simulink model "robot_simulation"  (R2025a)
settings: Solver=VariableStepAuto  StartTime=0.0  StopTime=50  FixedStep=0.01  MaxStep=0.1  RelTol=1e-3
settings Model: Creator=davrahnpaur  LastModifiedBy=davrahnpaur

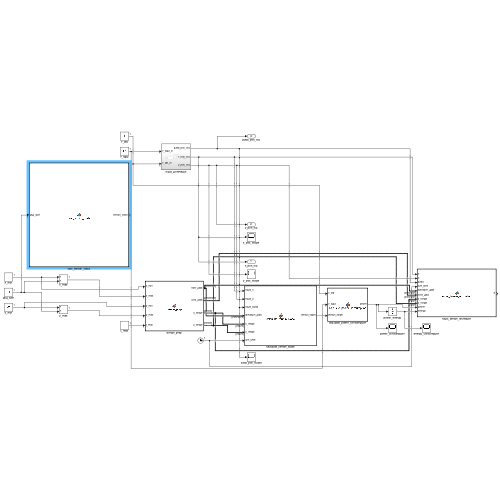
[thumbnail: Simulink's stored preview of the top-level diagram]
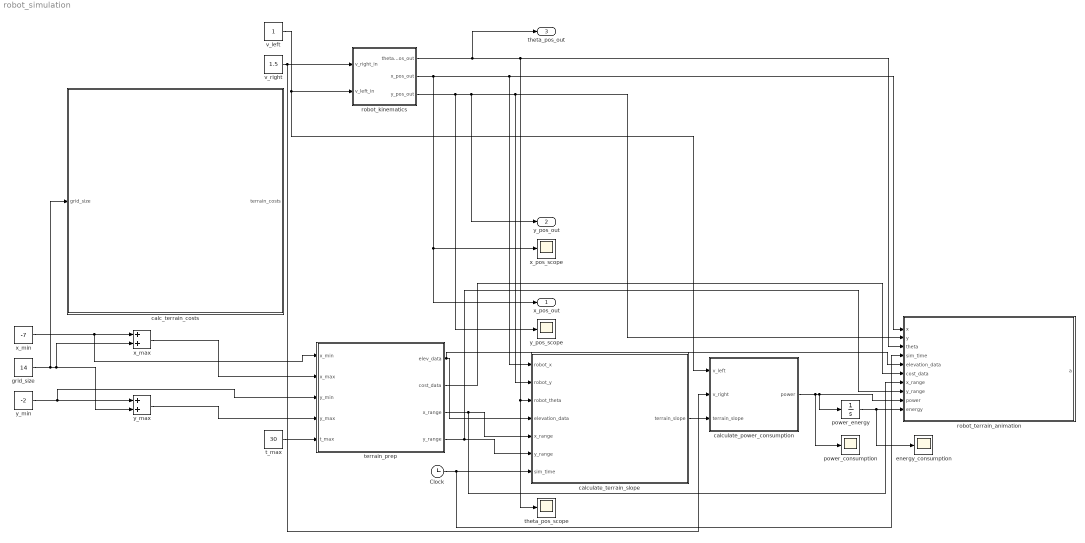
== system robot_simulation ==
  Clock : Clock
  calc_terrain_costs : MATLAB Function  TreatAsAtomicUnit=on
  calculate_power_consumption : MATLAB Function  TreatAsAtomicUnit=on
  calculate_terrain_slope : MATLAB Function  TreatAsAtomicUnit=on  SystemSampleTime=0.01
  energy_consumption : Scope
      settings: ActiveDisplayYMinimum=-15.735326881390064  ActiveDisplayYMaximum=141.6179419325106  DataLoggingVariableName=ScopeData4
  grid_size : Constant  Value=14
  power_consumption : Scope
      settings: ActiveDisplayYMinimum=1.5743115904386631  ActiveDisplayYMaximum=3.4296984826344525  DataLoggingVariableName=ScopeData3
  power_energy : Integrator
  robot_kinematics : Subsystem
  robot_terrain_animation : MATLAB Function  TreatAsAtomicUnit=on  SystemSampleTime=0.5
  t_max : Constant  Value=30
  terrain_prep : MATLAB Function  TreatAsAtomicUnit=on
  theta_pos_scope : Scope
      settings: ActiveDisplayYMinimum=-1  ActiveDisplayYMaximum=1
  v_left : Constant
  v_right : Constant  Value=1.5
  x_max : Sum
  x_min : Constant  Value=-7
  x_pos_scope : Scope
      settings: ActiveDisplayYMinimum=-1  ActiveDisplayYMaximum=1
  y_max : Sum
  y_min : Constant  Value=-2
  y_pos_scope : Scope
      settings: ActiveDisplayYMinimum=-1  ActiveDisplayYMaximum=1  DataLoggingVariableName=ScopeData2
  x_pos_out : Outport
  y_pos_out : Outport  Port=2
  theta_pos_out : Outport  Port=3
  wires:
  power_energy/1 -> robot_terrain_animation/10(energy), energy_consumption/1
  calculate_terrain_slope/1(terrain_slope) -> calculate_power_consumption/3(terrain_slope)
  calculate_power_consumption/1(power) -> power_energy/1, robot_terrain_animation/9(power), power_consumption/1
  Clock/1 -> calculate_terrain_slope/7(sim_time), robot_terrain_animation/4(sim_time)
  terrain_prep/4(y_range) -> calculate_terrain_slope/6(y_range), robot_terrain_animation/8(y_range)
  terrain_prep/3(x_range) -> calculate_terrain_slope/5(x_range), robot_terrain_animation/7(x_range)
  terrain_prep/2(cost_data) -> robot_terrain_animation/6(cost_data)
  terrain_prep/1(elev_data) -> calculate_terrain_slope/4(elevation_data), robot_terrain_animation/5(elevation_data)
  t_max/1 -> terrain_prep/5(t_max)
  robot_kinematics/3(y_pos_out) -> calculate_terrain_slope/2(robot_y), robot_terrain_animation/2(y), y_pos_out/1, y_pos_scope/1
  x_min/1 -> x_max/1, terrain_prep/1(x_min)
  robot_kinematics/1(theta_pos_out) -> calculate_terrain_slope/3(robot_theta), theta_pos_scope/1, robot_terrain_animation/3(theta), theta_pos_out/1
  x_max/1 -> terrain_prep/2(x_max)
  grid_size/1 -> y_max/2, x_max/2, calc_terrain_costs/1(grid_size)
  y_max/1 -> terrain_prep/4(y_max)
  v_right/1 -> robot_kinematics/1(v_right_in), calculate_power_consumption/2(v_right)
  robot_kinematics/2(x_pos_out) -> x_pos_out/1, x_pos_scope/1, calculate_terrain_slope/1(robot_x), robot_terrain_animation/1(x)
  y_min/1 -> y_max/1, terrain_prep/3(y_min)
  v_left/1 -> robot_kinematics/2(v_left_in), calculate_power_consumption/1(v_left)

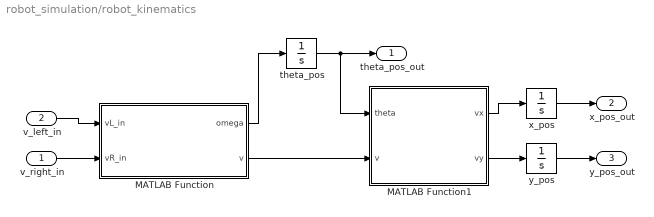
== system robot_simulation/robot_kinematics ==
  v_right_in : Inport
  v_left_in : Inport  Port=2
  MATLAB Function : MATLAB Function  TreatAsAtomicUnit=on
  MATLAB Function1 : MATLAB Function  TreatAsAtomicUnit=on
  theta_pos : Integrator
  x_pos : Integrator  ContinuousStateAttributes='x_position'
  y_pos : Integrator  ContinuousStateAttributes='y_position'
  theta_pos_out : Outport
  x_pos_out : Outport  Port=2
  y_pos_out : Outport  Port=3
  wires:
  x_pos/1 -> x_pos_out/1
  MATLAB Function1/2(vy) -> y_pos/1
  MATLAB Function1/1(vx) -> x_pos/1
  v_left_in/1 -> MATLAB Function/1(vL_in)
  v_right_in/1 -> MATLAB Function/2(vR_in)
  theta_pos/1 -> MATLAB Function1/1(theta), theta_pos_out/1
  y_pos/1 -> y_pos_out/1
  MATLAB Function/2(v) -> MATLAB Function1/2(v)
  MATLAB Function/1(omega) -> theta_pos/1

== matlab function robot_simulation/robot_kinematics/MATLAB Function ==
  data: vL_in input; omega output; vR_in input; v output
function [omega,v] = velocity_transform(vL_in,vR_in)

    omega = (vR_in-vL_in)/2;
    v = (vR_in+vL_in)/2;
end

== matlab function robot_simulation/robot_terrain_animation ==
  data: x input; y input; theta input; a output; sim_time input; elevation_data input; cost_data input; x_range input; y_range input; power input; energy input
function a = robot_terrain_animation(x, y, theta, sim_time, elevation_data, cost_data, x_range, y_range, power, energy)
%#codegen
    persistent trail_x trail_y X_grid Y_grid
    
    % Initialize grid (do once)
    if isempty(X_grid)
        [X_grid, Y_grid] = meshgrid(x_range, y_range);
        trail_x = [];
        trail_y = [];
    end
    
    % Calculate current terrain time slice
    time_index = max(1, min(sim_time+1, size(elevation_data,3)));
    current_elevation = elevation_data(:,:,time_index);
    current_cost = cost_data(:,:,time_index);
    
    % Clear and redraw
    cla;
    
    % Draw terrain background
    % Cost as heatmap background
    imagesc(x_range, y_range, current_cost);
    hold on;
    
    % Elevation as contour lines
    contour(x_range, y_range, current_elevation, 'k-', 'LineWidth', 0.5);
    
    % Your existing robot visualization
    plot(x, y, 'ro', 'MarkerSize', 10, 'MarkerFaceColor', 'red');
    
    % Robot heading arrow
    arrow_length = 0.5;
    arrow_x = [x, x + arrow_length*cos(theta)];
    arrow_y = [y, y + arrow_length*sin(theta)];
    plot(arrow_x, arrow_y, 'b-', 'LineWidth', 3);
    
    % Trail
    trail_x = [trail_x, x];
    trail_y = [trail_y, y];
    plot(trail_x, trail_y, 'g--', 'LineWidth', 2);
    
    % Formatting
    axis equal;
    xlim([x_range(1), x_range(end)]);
    ylim([y_range(1), y_range(end)]);
    colorbar;  % Show cost scale
    title(sprintf('Time: %.1f s | Power: %.1f W | Energy: %.1f J', sim_time, power, energy));
    
    drawnow;
    a = 0;
end

== matlab function robot_simulation/robot_kinematics/MATLAB Function1 ==
  data: theta input; vx output; v input; vy output
function [vx,vy] = velocity_transform2(theta,v)
   vx = v*cos(theta);
   vy = v*sin(theta);
end

== matlab function robot_simulation/terrain_prep ==
  data: elev_data output; cost_data output; x_range output; y_range output; x_min input; x_max input; y_min input; y_max input; t_max input
function [elev_data, cost_data, x_range, y_range] = terrain_prep(x_min,x_max,y_min,y_max,t_max)
    % Define spatial grid - these should match your animation axis limits
    num_x = (x_max - x_min) + 1;
    num_y = (y_max - y_min) + 1;
    x_range = linspace(x_min, x_max, num_x);
    y_range = linspace(y_min, y_max, num_y);
    
    % Time parameters
    time_steps = t_max + 1;  % Number of terrain snapshots
    
    % Initialize terrain arrays
    elev_data = zeros(length(y_range), length(x_range), time_steps);
    cost_data = zeros(length(y_range), length(x_range), time_steps);
    
    % Create example terrain that changes over time
    [x_grid, y_grid] = meshgrid(x_range, y_range);
    
    for t = 1:time_steps
        time_factor = t-1;
        
        % Example elevation: moving sine wave
        elev_data(:,:,t) = 2 * sin(0.3 * x_grid + 0.1 * time_factor) .* cos(0.2 * y_grid);
        
        % Example cost: moving high-cost regions
        cost_data(:,:,t) = 1 + 2 * exp(-((x_grid - 5 - time_factor/3).^2 + (y_grid - 2).^2) / 4);
    end
end

== matlab function robot_simulation/calculate_power_consumption ==
  data: v_left input; power output; v_right input; terrain_slope input
function power = calculate_power_consumption(v_left, v_right, terrain_slope)

    % Base power consumption (flat terrain)
    base_power_left = abs(v_left);% * 10;   % 10 watts per m/s
    base_power_right = abs(v_right);% * 10; % 10 watts per m/s
    
    % Slope effect multiplier
    % Positive slope (uphill) increases power, negative (downhill) decreases it
    slope_multiplier = 1 + terrain_slope * 0.5;  % 50% more power per unit slope
    slope_multiplier = max(0.1, slope_multiplier); % Minimum 10% power (even downhill)
    
    % Total power consumption
    power = (base_power_left + base_power_right) * slope_multiplier;

end

== matlab function robot_simulation/calc_terrain_costs ==
  data: grid_size input; terrain_costs output
function terrain_costs = calc_terrain_costs(grid_size)
    % Define grid dimensions
    
    % Define terrain types and their properties, INCLUDING COSTS
    terrain_types = {
        struct('name', 'Grass', 'color', [0.3 0.6 0.2], 'cost', 1.0);     % Green, low cost
        struct('name', 'Sand', 'color', [0.9 0.8 0.5], 'cost', 2.0);      % Light Brown/Yellow, moderate cost
        struct('name', 'Mud', 'color', [0.5 0.3 0.1], 'cost', 3.0);       % Dark Brown, higher cost
        struct('name', 'Road', 'color', [0.6 0.6 0.6], 'cost', 0.5);      % Grey, very low cost (fast)
        struct('name', 'Water', 'color', [0.2 0.4 0.8], 'cost', inf);     % Blue, impassable
        struct('name', 'Forest', 'color', [0.1 0.4 0.1], 'cost', 2.5);    % Darker Green, moderate-high cost
    };
    num_terrain_types = length(terrain_types);
    
    terrain_grid = zeros(grid_size, grid_size);
    
    % --- Initial Random Terrain Generation ---
    % Assign a random terrain type to each cell in the grid
    for i = 1:grid_size
        for j = 1:grid_size
            terrain_grid(i, j) = randi(num_terrain_types);
        end
    end
    
    % --- Terrain Smoothing (to create grouped regions) ---
    num_smoothing_iterations = 5;
    for iter = 1:num_smoothing_iterations
        new_terrain_grid = terrain_grid; % Create a copy to store updates for this iteration
        for i = 1:grid_size
            for j = 1:grid_size
                neighbors = [];
                % Check 8-directional neighbors
                for dx = -1:1
                    for dy = -1:1
                        if dx == 0 && dy == 0
                            continue; % Skip the current cell itself
                        end
                        ni = i + dx;
                        nj = j + dy;
                        % Check if neighbor is within grid bounds
                        if ni >= 1 && ni <= grid_size && nj >= 1 && nj <= grid_size
                            neighbors = [neighbors, terrain_grid(ni, nj)];
                        end
                    end
                end
    
                % If the cell has neighbors, find the most frequent terrain type among them
                if ~isempty(neighbors)
                    unique_neighbors = unique(neighbors);
                    counts = zeros(1, length(unique_neighbors));
                    for k = 1:length(unique_neighbors)
                        counts(k) = sum(neighbors == unique_neighbors(k));
                    end
                    [~, max_idx] = max(counts);
                    most_frequent_terrain = unique_neighbors(max_idx);
                    new_terrain_grid(i, j) = most_frequent_terrain;
                end
            end
        end
        terrain_grid = new_terrain_grid;
    end
    
    terrain_costs = terrain_grid;
end

== matlab function robot_simulation/calculate_terrain_slope ==
  data: robot_x input; terrain_slope output; robot_y input; robot_theta input; elevation_data input; x_range input; y_range input; sim_time input
function terrain_slope = calculate_terrain_slope(robot_x, robot_y, robot_theta, elevation_data, x_range, y_range, sim_time)
    
    time_index = round(max(1, min(sim_time+1, size(elevation_data,3))));
    % Find robot position in grid coordinates
    x_idx = max(1, min(length(x_range), round((robot_x - x_range(1)) / (x_range(2) - x_range(1))) + 1));
    y_idx = max(1, min(length(y_range), round((robot_y - y_range(1)) / (y_range(2) - y_range(1))) + 1));
    
    % Get current elevation (use first time slice for now)
    current_elevation = elevation_data(:,:,time_index);
    
    % Calculate gradient (slope) at robot position
    dx = x_range(2) - x_range(1);
    dy = y_range(2) - y_range(1);
    
    % Get neighboring elevation points for gradient calculation
    if x_idx < length(x_range) && y_idx < length(y_range)
        % Elevation gradient in x and y directions
        grad_x = (current_elevation(y_idx, x_idx+1) - current_elevation(y_idx, x_idx)) / dx;
        grad_y = (current_elevation(y_idx+1, x_idx) - current_elevation(y_idx, x_idx)) / dy;
        
        % Slope in robot's heading direction
        terrain_slope = grad_x * cos(robot_theta) + grad_y * sin(robot_theta);
    else
        terrain_slope = 0;  % Default to flat if at boundary
    end

end
